simulink model "model2"  (Simulink 6.6)
settings: Solver=ode45  StartTime=0.0  StopTime=12  RelTol=1e-3
settings Model: Creator=mxkana  LastModifiedBy=mxkana

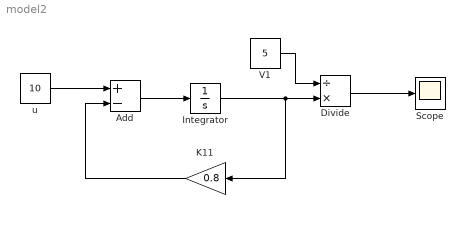
== system model2 ==
  Add : Sum  Inputs=+-  OutScaling=2^-10
  Divide : Product  Inputs=/*  OutScaling=2^-10
  Integrator : Integrator
  K11 : Gain  Orientation=left  Gain=0.8
  Scope : Scope
  V1 : Constant  Value=5
  u : Constant  Value=10
  wires:
  Integrator/1 -> K11/1, Divide/2
  K11/1 -> Add/2
  V1/1 -> Divide/1
  Divide/1 -> Scope/1
  Add/1 -> Integrator/1
  u/1 -> Add/1
